simulink model "task9"  (R2023a)
settings: Solver=VariableStepAuto  StartTime=0.0  StopTime=10.0  RelTol=1e-3
undefined symbols (not defined in the file or in its folder): VirtualWallLogic
libraries: simulink x2
settings Model: Creator=LENOVO  LastModifiedBy=LENOVO

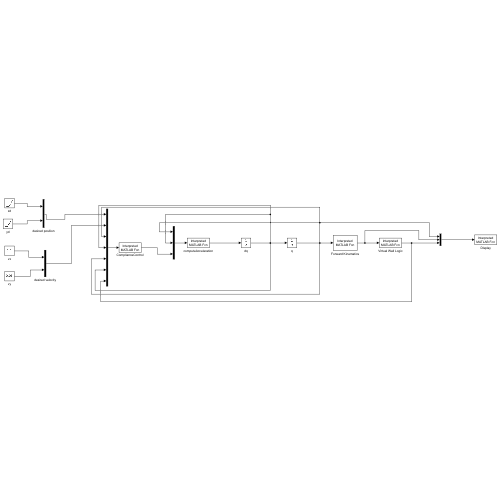
[thumbnail: Simulink's stored preview of the top-level diagram]
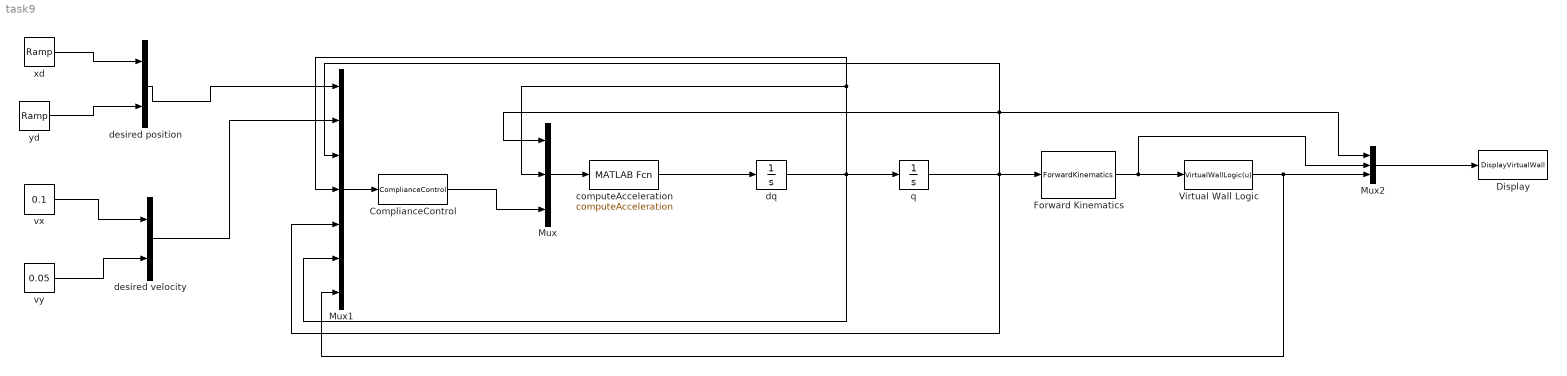
== system task9 ==
  ComplianceControl : MATLABFcn  MATLABFcn=ComplianceControl  OutputDimensions=2
  Display : MATLABFcn  MATLABFcn=DisplayVirtualWall  OutputDimensions=0
  Forward Kinematics : MATLABFcn  MATLABFcn=ForwardKinematics  OutputDimensions=2  Output1D=off
  Mux : Mux  Inputs=3
  Mux1 : Mux  Inputs=7
  Mux2 : Mux  Inputs=3
  Virtual Wall Logic : MATLABFcn  MATLABFcn=VirtualWallLogic(u)  OutputDimensions=2
  computeAcceleration : MATLABFcn  MATLABFcn=computeAcceleration  OutputDimensions=2  Output1D=off
  desired position : Mux  Inputs=2
  desired velocity : Mux  Inputs=2
  dq : Integrator  InitialCondition=[0; 0]
  q : Integrator  InitialCondition=[pi/2; pi/4]
  vx : Constant  Value=0.1
  vy : Constant  Value=0.05
  xd : simulink/Sources/Ramp  slope=0.1  start=0  InitialOutput=0
  yd : simulink/Sources/Ramp  slope=0.05  start=0  InitialOutput=0
  wires:
  ComplianceControl/1 -> Mux/3
  yd/1 -> desired position/2
  desired position/1 -> Mux1/1
  desired velocity/1 -> Mux1/2
  vx/1 -> desired velocity/1
  Mux1/1 -> ComplianceControl/1
  vy/1 -> desired velocity/2
  Mux/1 -> computeAcceleration/1
  dq/1 -> Mux1/6, Mux1/4, Mux/2, q/1
  computeAcceleration/1 -> dq/1
  xd/1 -> desired position/1
  Forward Kinematics/1 -> Mux2/2, Virtual Wall Logic/1
  Virtual Wall Logic/1 -> Mux2/3, Mux1/7
  q/1 -> Mux1/5, Forward Kinematics/1, Mux2/1, Mux1/3, Mux/1
  Mux2/1 -> Display/1
